simulink model "ortho_CAN_controlV2"  (R2016b)
settings: Solver=FixedStepDiscrete  StartTime=0.0  StopTime=180  FixedStep=.001  RelTol=1e-3  EnableMultiTasking=on
values from neighbouring files (symbols this model uses):
  rho1 = (rho01*(1-d(3)))+(rho11*d(3))    [fcn.m]
  rho2 = (rho02*(1-d(3)))+(rho12*d(3))    [fcn.m]
  theta1 = (theta01*(1-d(3)))+(theta11*d(3))    [fcn.m]
  theta2 = (theta02*(1-d(3)))+(theta12*d(3))    [fcn.m]
undefined symbols (not defined in the file or in its folder): bit, fdesignblkfcn, gcbh, rho_end, Standard, theta_end
libraries: slrtlib x7, simulink x6, slrtsoftinglib x3, xpcnilib x3, canmsglib x2
(part 2 of 2)

== matlab function ortho_CAN_controlV2/Subsystem/MATLAB Function ==
  data: pos input; vel input; unused input; unused1 input; r1 input; t1 input; r2 input; t2 input; r3 input; t3 input; r4 input; t4 input; rho output; theta output; segin input; i input; iout output; ti input; to output; time input
function [rho,theta,iout,to] = fcn(pos,vel,~,~,r1,t1,r2,t2,r3,t3,r4,t4,segin,i,ti,time)
%#codegen

p=pos./10;
v=vel;
% iout=i;
% to=ti;
% rho=0;
% theta=0;

%TRILINEAR INTERPOLATION
    %set upper and lower map points
    up=ceil(p);
    low=floor(p);
    %determine distance from current point to lower map point
    d=p-low;
    
    rho001=(r1(low(1),low(2),low(3))*(1-d(1)))+(r1(up(1),low(2),low(3))*d(1));
    theta001=(t1(low(1),low(2),low(3))*(1-d(1)))+(t1(up(1),low(2),low(3))*d(1));
    rho101=(r1(low(1),up(2),low(3))*(1-d(1)))+(r1(up(1),up(2),low(3))*d(1));
    theta101=(t1(low(1),up(2),low(3))*(1-d(1)))+(t1(up(1),up(2),low(3))*d(1));
    rho011=(r1(low(1),low(2),up(3))*(1-d(1)))+(r1(up(1),low(2),up(3))*d(1));
    theta011=(t1(low(1),low(2),up(3))*(1-d(1)))+(t1(up(1),low(2),up(3))*d(1));
    rho111=(r1(low(1),up(2),up(3))*(1-d(1)))+(r1(up(1),up(2),up(3))*d(1));
    theta111=(t1(low(1),up(2),up(3))*(1-d(1)))+(t1(up(1),up(2),up(3))*d(1));
    rho01=(rho001*(1-d(2)))+(rho101*d(2));
    theta01=(theta001*(1-d(2)))+(theta101*d(2));
    rho11=(rho011*(1-d(2)))+(rho111*d(2));
    theta11=(theta011*(1-d(2)))+(theta111*d(2));
    rho1=(rho01*(1-d(3)))+(rho11*d(3));
    theta1=(theta01*(1-d(3)))+(theta11*d(3));
    
    
    rho002=(r2(low(1),low(2),low(3))*(1-d(1)))+(r2(up(1),low(2),low(3))*d(1));
    theta002=(t2(low(1),low(2),low(3))*(1-d(1)))+(t2(up(1),low(2),low(3))*d(1));
    rho102=(r2(low(1),up(2),low(3))*(1-d(1)))+(r2(up(1),up(2),low(3))*d(1));
    theta102=(t2(low(1),up(2),low(3))*(1-d(1)))+(t2(up(1),up(2),low(3))*d(1));
    rho012=(r2(low(1),low(2),up(3))*(1-d(1)))+(r2(up(1),low(2),up(3))*d(1));
    theta012=(t2(low(1),low(2),up(3))*(1-d(1)))+(t2(up(1),low(2),up(3))*d(1));
    rho112=(r2(low(1),up(2),up(3))*(1-d(1)))+(r2(up(1),up(2),up(3))*d(1));
    theta112=(t2(low(1),up(2),up(3))*(1-d(1)))+(t2(up(1),up(2),up(3))*d(1));
    rho02=(rho002*(1-d(2)))+(rho102*d(2));
    theta02=(theta002*(1-d(2)))+(theta102*d(2));
    rho12=(rho012*(1-d(2)))+(rho112*d(2));
    theta12=(theta012*(1-d(2)))+(theta112*d(2));
    rho2=(rho02*(1-d(3)))+(rho12*d(3));
    theta2=(theta02*(1-d(3)))+(theta12*d(3));
     
    rho003=(r3(low(1),low(2),low(3))*(1-d(1)))+(r3(up(1),low(2),low(3))*d(1));
    theta003=(t3(low(1),low(2),low(3))*(1-d(1)))+(t3(up(1),low(2),low(3))*d(1));
    rho103=(r3(low(1),up(2),low(3))*(1-d(1)))+(r3(up(1),up(2),low(3))*d(1));
    theta103=(t3(low(1),up(2),low(3))*(1-d(1)))+(t3(up(1),up(2),low(3))*d(1));
    rho013=(r3(low(1),low(2),up(3))*(1-d(1)))+(r3(up(1),low(2),up(3))*d(1));
    theta013=(t3(low(1),low(2),up(3))*(1-d(1)))+(t3(up(1),low(2),up(3))*d(1));
    rho113=(r3(low(1),up(2),up(3))*(1-d(1)))+(r3(up(1),up(2),up(3))*d(1));
    theta113=(t3(low(1),up(2),up(3))*(1-d(1)))+(t3(up(1),up(2),up(3))*d(1));
    rho03=(rho003*(1-d(2)))+(rho103*d(2));
    theta03=(theta003*(1-d(2)))+(theta103*d(2));
    rho13=(rho013*(1-d(2)))+(rho113*d(2));
    theta13=(theta013*(1-d(2)))+(theta113*d(2));
    rho3=(rho03*(1-d(3)))+(rho13*d(3));
    theta3=(theta03*(1-d(3)))+(theta13*d(3));
    
%     rho004=(r4(low(1),low(2),low(3))*(1-d(1)))+(r4(up(1),low(2),low(3))*d(1));
%     theta004=(t4(low(1),low(2),low(3))*(1-d(1)))+(t4(up(1),low(2),low(3))*d(1));
%     rho104=(r4(low(1),up(2),low(3))*(1-d(1)))+(r4(up(1),up(2),low(3))*d(1));
%     theta104=(t4(low(1),up(2),low(3))*(1-d(1)))+(t4(up(1),up(2),low(3))*d(1));
%     rho014=(r4(low(1),low(2),up(3))*(1-d(1)))+(r4(up(1),low(2),up(3))*d(1));
%     theta014=(t4(low(1),low(2),up(3))*(1-d(1)))+(t4(up(1),low(2),up(3))*d(1));
%     rho114=(r4(low(1),up(2),up(3))*(1-d(1)))+(r4(up(1),up(2),up(3))*d(1));
%     theta114=(t4(low(1),up(2),up(3))*(1-d(1)))+(t4(up(1),up(2),up(3))*d(1));
%     rho04=(rho004*(1-d(2)))+(rho104*d(2));
%     theta04=(theta004*(1-d(2)))+(theta104*d(2));
%     rho14=(rho014*(1-d(2)))+(rho114*d(2));
%     theta14=(theta014*(1-d(2)))+(theta114*d(2));
%     rho4=(rho04*(1-d(3)))+(rho14*d(3));
%     theta4=(theta04*(1-d(3)))+(theta14*d(3));
% 
%     rho005=(r5(low(1),low(2),low(3))*(1-d(1)))+(r5(up(1),low(2),low(3))*d(1));
%     theta005=(t5(low(1),low(2),low(3))*(1-d(1)))+(t5(up(1),low(2),low(3))*d(1));
%     rho105=(r5(low(1),up(2),low(3))*(1-d(1)))+(r5(up(1),up(2),low(3))*d(1));
%     theta105=(t5(low(1),up(2),low(3))*(1-d(1)))+(t5(up(1),up(2),low(3))*d(1));
%     rho015=(r5(low(1),low(2),up(3))*(1-d(1)))+(r5(up(1),low(2),up(3))*d(1));
%     theta015=(t5(low(1),low(2),up(3))*(1-d(1)))+(t5(up(1),low(2),up(3))*d(1));
%     rho115=(r5(low(1),up(2),up(3))*(1-d(1)))+(r5(up(1),up(2),up(3))*d(1));
%     theta115=(t5(low(1),up(2),up(3))*(1-d(1)))+(t5(up(1),up(2),up(3))*d(1));
%     rho05=(rho005*(1-d(2)))+(rho105*d(2));
%     theta05=(theta005*(1-d(2)))+(theta105*d(2));
%     rho15=(rho015*(1-d(2)))+(rho115*d(2));
%     theta15=(theta015*(1-d(2)))+(theta115*d(2));
%     rho5=(rho05*(1-d(3)))+(rho15*d(3));
%     theta5=(theta05*(1-d(3)))+(theta15*d(3));
    
%% CUP TASK
%     if segin(i) == 1
%         if p(2) >= 35 && p(3) >= 15
%             if v > -1e-2 %&& abs(v(2)) <= 5
%                 iout=i+1;
%                 to=time+.4;
%             else 
%                 iout=i;
%                 to=ti;
%             end
%         else
%             iout=i;
%             to=ti;
%         end
%         rho=(1./(1+exp(-(time-ti)./.058)))*rho1;
%         theta=(1./(1+exp(-(time-ti)./.058)))*theta1;
%         
%     elseif segin(i) == 2
%         if p(1) <= 34 && p(2) <= 27.5
%             iout=1;
%             to=time+.4;
%         else
%             iout=i;
%             to=ti;
%         end
%         rho=((1-(1./(1+exp(-(time-ti)./.058))))*rho1)+((1./(1+exp(-(time-ti)./.058)))*rho2);
%         theta=((1-(1./(1+exp(-(time-ti)./.058))))*theta1)+((1./(1+exp(-(time-ti)./.058)))*theta2);
% %         rho=rho2;
% %         theta=theta2;
%         
%     else 
%         rho=((1-(1./(1+exp(-(time-ti)./.058))))*rho2);
%         theta=((1-(1./(1+exp(-(time-ti)./.058))))*theta2);
% %         theta=0;
%         if p(1) >= 34 %&& p(2) <= 22
%             iout=i+1;
%             to=time+.4;
%         else
%             iout=i;
%             to=ti;
%         end 
%         
%     end

%% PITCHER TASK
%     if segin(i) == 1
%         if p(1) >= 46 && p(3) >= 18
%             if v > -1e-2 %&& abs(v(2)) <= 5
%                 iout=i+1;
%                 to=time+.4;
%             else 
%                 iout=i;
%                 to=ti;
%             end
%         else
%             iout=i;
%             to=ti;
%         end
%         rho=(1./(1+exp(-(time-ti)./.058)))*rho1;
%         theta=(1./(1+exp(-(time-ti)./.058)))*theta1;
%     
%     elseif segin(i) == 2
%         if p(1) <= 34 && p(2) <= 27.5
%             iout=1;
%             to=time+.4;
%         else
%             iout=i;
%             to=ti;
%         end
%         rho=((1-(1./(1+exp(-(time-ti)./.058))))*rho1)+((1./(1+exp(-(time-ti)./.058)))*rho2);
%         theta=((1-(1./(1+exp(-(time-ti)./.058))))*theta1)+((1./(1+exp(-(time-ti)./.058)))*theta2);
%       
%     else 
%         rho=((1-(1./(1+exp(-(time-ti)./.058))))*rho2);
%         theta=((1-(1./(1+exp(-(time-ti)./.058))))*theta2);
%         if p(1) >= 34 %&& p(2) <= 22
%             iout=i+1;
%             to=time+.4;
%         else
%             iout=i;
%             to=ti;
%         end 
%       
%     end
%% SPOON TASK
    if segin(i) == 1
        if p(2) >= 35 && p(3) >= 18
            if v > -1e-2 %&& abs(v(2)) <= 5
                iout=i+1;
                to=time+.4;
            else 
                iout=i;
                to=ti;
            end
        else
            iout=i;
            to=ti;
        end
        rho=(1./(1+exp(-(time-ti)./.058)))*rho1;
        theta=(1./(1+exp(-(time-ti)./.058)))*theta1;
        
    elseif segin(i) == 2
        if p(1) <= 34 && p(2) <= 27.5
            iout=1;
            to=time+.4;
        else
            iout=i;
            to=ti;
        end
        rho=((1-(1./(1+exp(-(time-ti)./.058))))*rho1)+((1./(1+exp(-(time-ti)./.058)))*rho2);%
        theta=((1-(1./(1+exp(-(time-ti)./.058))))*theta1)+((1./(1+exp(-(time-ti)./.058)))*theta2);
          
    else 
        rho=((1-(1./(1+exp(-(time-ti)./.058))))*rho2);
        theta=((1-(1./(1+exp(-(time-ti)./.058))))*theta2);
        if p(1) >= 34 %&& p(2) <= 22
            iout=i+1;
            to=time+.4;
        else
            iout=i;
            to=ti;
        end 
        
    end
%% CONE TASK
%     if segin(i) == 1
%         if p(2) <= 24 
%             if abs(v(2)) < 20 %&& abs(v(2)) <= 5
%                 iout=i+1;
%                 to=time+.4;
%             else 
%                 iout=i;
%                 to=ti;
%             end
%         else
%             iout=i;
%             to=ti;
%         end
%         rho=(1./(1+exp(-(time-ti)./.058)))*rho1;
%         theta=(1./(1+exp(-(time-ti)./.058)))*theta1;
%         rho=rho1;
%         theta=theta1;
%     if segin(i) == 1
%         if p(1) >= 45
%             if abs(v(1)) < 20
%                 iout=i+1;
%                 to=time+.4;
%             else
%                 iout=i;
%                 to=ti;
%             end
%         else
%             iout=i;
%             to=ti;
%         end
%         if segin(i-1) == 9
%             rho=((1-(1./(1+exp(-(time-ti)./.058))))*rho1)+((1./(1+exp(-(time-ti)./.058)))*rho2);
%             theta=((1-(1./(1+exp(-(time-ti)./.058))))*theta1)+((1./(1+exp(-(time-ti)./.058)))*theta2);
%             rho=(1./(1+exp(-(time-ti)./.058)))*rho1;
%             theta=(1./(1+exp(-(time-ti)./.058)))*theta1;
%         else
%             rho=((1-(1./(1+exp(-(time-ti)./.058))))*rho2)+((1./(1+exp(-(time-ti)./.058)))*rho1);
%             theta=((1-(1./(1+exp(-(time-ti)./.058))))*theta2)+((1./(1+exp(-(time-ti)./.058)))*theta1);
%         end
%     elseif segin(i) == 2
%         if p(1) <= 40
%             if abs(v(1)) < 20
%                 iout=i+1;
%                 to=time+.4;
%             else
%                 iout=i;
%                 to=ti;
%             end
%         else
%             iout=i;
%             to=ti;
%         end
%         rho=((1-(1./(1+exp(-(time-ti)./.058))))*rho1)+((1./(1+exp(-(time-ti)./.058)))*rho2);
%         theta=((1-(1./(1+exp(-(time-ti)./.058))))*theta1)+((1./(1+exp(-(time-ti)./.058)))*theta2);
%     elseif segin(i) == 3
%         if p(1) <= 34 && p(2) <= 27.5 
%             iout=1;
%             to=time+.4;
%         else
%             iout=i;
%             to=ti;
%         end
%         rho=((1-(1./(1+exp(-(time-ti)./.058))))*rho1)+((1./(1+exp(-(time-ti)./.058)))*rho3);
%         theta=((1-(1./(1+exp(-(time-ti)./.058))))*theta1)+((1./(1+exp(-(time-ti)./.058)))*theta3);
%     else 
%         rho=((1-(1./(1+exp(-(time-ti)./.058))))*rho3);
%         theta=((1-(1./(1+exp(-(time-ti)./.058))))*theta3);
%         if p(1) >= 34 %&& p(2) <= 22
%             iout=i+1;
%             to=time+.4;
%         else
%             iout=i;
%             to=ti;
%         end 
%         rho=0;
%         theta=0;
%     end
%% PEG TASK
% 
% if segin(i) == 1
%     if p(1) >= 47.5 && p(2) <= 12 && p(3) >= 10
%         if v < 1e-2
%             iout=i+1;
%             to=time+.4;
%         else
%             iout=i;
%             to=ti;
%         end
%     else
%         iout=i;
%         to=ti;
%     end
%     rho=(1./(1+exp(-(time-ti)./.058)))*rho1;
%     theta=(1./(1+exp(-(time-ti)./.058)))*theta1;
% elseif segin(i) == 2
%     if p(1) <= 34 && p(2) <= 27.5
%         iout=1;
%         to=time+.4;
%     else
%         iout=i;
%         to=ti;
%     end
%     rho=((1-(1./(1+exp(-(time-ti)./.058))))*rho1)+((1./(1+exp(-(time-ti)./.058)))*rho2);
%     theta=((1-(1./(1+exp(-(time-ti)./.058))))*theta1)+((1./(1+exp(-(time-ti)./.058)))*theta2);
% else
%     if p(1) >= 34 && p(2) <= 22
%         iout=i+1;
%         to=time+.4;
%     else
%         iout=i;
%         to=ti;
%     end
%     rho=((1-(1./(1+exp(-(time-ti)./.058))))*rho2);
%     theta=((1-(1./(1+exp(-(time-ti)./.058))))*theta2);
% end

== matlab function ortho_CAN_controlV2/Data Acq/forward kinematics ==
  data: x output; j1 input; y output; j2 input; d3 input; j4 input; j5 input; j6 input; z output
function [x,y,z] = fcn(j1,j2,d3,j4,j5,j6)
%#codegen

d1=336.55;
%a2=434.46; %original distance from x2 to x4 when arm is fully retracted
a2=406.4; %new distance from x2 to x4 when arm is fully retracted
d4=45.86;
a5=120.51;
d6=67.08;
a6=39.52;

s1=sind(j1);
c1=cosd(j1);
s2=sind(j2);
c2=cosd(j2);
s4=sind(j4);
c4=cosd(j4);
s5=sind(j5);
c5=cosd(j5);
s6=sind(j6);
c6=cosd(j6);

x = -a6*c6*((c1*s2*c5)+s5*((s1*c4)-(c1*c2*s4)))+a6*s6*((s1*s4)+(c1*c2*c4))-d6*((c1*s2*s5)-c5*((s1*c4)-(c1*c2*s4)))-(a5*c1*s2*c5)-a5*s5*((s1*c4)-(c1*c2*s4))-(d4*c1*s2)+((a2+d3)*c1*c2);
y = -a6*c6*((s1*s2*c5)-s5*((c1*c4)+(s1*c2*s4)))-a6*s6*((c1*s4)-(s1*c2*c4))-d6*((s1*s2*s5)+c5*((c1*c4)+(s1*c2*s4)))-(a5*s1*s2*c5)+a5*s5*((c1*c4)+(s1*c2*s4))-(d4*s1*s2)+((a2+d3)*s1*c2);
z = -a6*c6*((c2*c5)+(s2*s4*s5))-(a6*s2*c4*s6)-d6*((c2*s5)-(s2*s4*c5))-(a5*c2*c5)-(a5*s2*s4*s5)-(d4*c2)-((a2+d3)*s2)+d1;
